simulink model "MyMotor_RTW"  (Simulink 10.1)
settings: Solver=ode1  StartTime=0.0  StopTime=inf  FixedStep=0.0002  RelTol=1e-3
PreLoadFcn:
  | vehicle = 'Car'; if ~length(which('cmcmd')), cmenv; end
  | MyMotor_RTW_bus
InitFcn:
  | vehicle = 'Car'; if ~length(which('cmcmd')), cmenv; end
  | MyMotor_RTW_bus
libraries: simulink x1, CarMaker4SL x1
Description:
  | CarMaker Plug-in Model Target
settings Model: Creator=ml  LastModifiedBy=ml
settings DataIOCC: LimitDataPoints=on  SignalLoggingSaveFormat=ModelDataLogs
settings OptimizationCC: ExpressionDepthLimit=2147483647
settings DebuggingCC: FcnCallInpInsideContextMsg=warning  StateNameClashWarn=warning  SFExecutionAtInitializationDiag=warning
settings HardwareCC: TargetHWDeviceType=32-bit Generic  ProdEqTarget=off
settings RTWCC: Description=CarMaker Plug-in Model Target  SystemTargetFile=CarMaker.tlc  TemplateMakefile=CarMaker_unix-win64.tmf
settings CodeAppCC: MaxIdLength=63
settings STFCustomTargetCC: ModelReferenceCompliant=off  MultiInstanceERTCode=on  CodeInterfacePackaging=Reusable function  CPPClassGenCompliant=on  GRTInterface=off  GenerateAllocFcn=on  SystemTargetFile=CarMaker.tlc
settings GRTTargetCC: ModelReferenceCompliant=off  ParMdlRefBuildCompliant=off  CompOptLevelCompliant=off  ConcurrentExecutionCompliant=off  MatFileLogging=off  MultiInstanceERTCode=on  CodeInterfacePackaging=Reusable function  GRTInterface=off  GenerateAllocFcn=on  UseToolchainInfoCompliant=off  ExtModeMexFile=noextcomm
settings CustomProperty: DataType=string
settings EnumStrPairs: String=Car

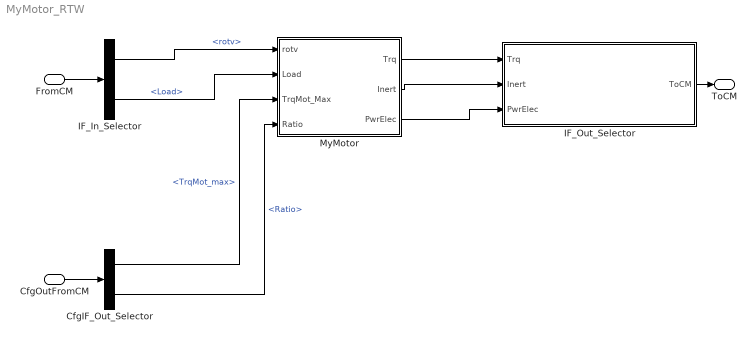
== system MyMotor_RTW ==
  FromCM : Inport  OutDataTypeStr=Bus: cmPTMotorIn
  CfgOutFromCM : Inport  Port=2  OutDataTypeStr=Bus: cmPTMotorCfgOut
  CfgIF_Out_Selector : BusSelector  OutputSignals=TrqMot_max,Ratio
  IF_In_Selector : BusSelector  OutputSignals=rotv,Load
  IF_Out_Selector : Subsystem  mask(Signal Selection){}
      mask help: Signal Selection Block
      settings: OpenFcn=cmSignalSelect('SignalSelection_CB',gcb)
  MyMotor : Subsystem
  ToCM : Outport  OutDataTypeStr=Bus: cmPTMotorOut  VectorParamsAs1DForOutWhenUnconnected=off
  wires:
  FromCM/1 -> IF_In_Selector/1
  IF_Out_Selector/1(ToCM) -> ToCM/1
  CfgOutFromCM/1 -> CfgIF_Out_Selector/1
  CfgIF_Out_Selector/1 -> MyMotor/3(TrqMot_Max)  "<TrqMot_max>"
  MyMotor/1(Trq) -> IF_Out_Selector/1(Trq)
  MyMotor/2(Inert) -> IF_Out_Selector/2(Inert)
  MyMotor/3(PwrElec) -> IF_Out_Selector/3(PwrElec)
  CfgIF_Out_Selector/2 -> MyMotor/4(Ratio)  "<Ratio>"
  IF_In_Selector/1 -> MyMotor/1(rotv)  "<rotv>"
  IF_In_Selector/2 -> MyMotor/2(Load)  "<Load>"

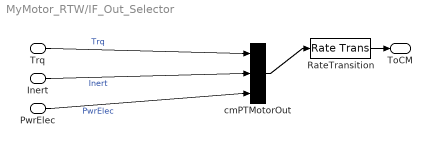
== system MyMotor_RTW/IF_Out_Selector ==
  Trq : Inport
  Inert : Inport  Port=2
  PwrElec : Inport  Port=3
  RateTransition : RateTransition  OutPortSampleTime=str2num(get_param(bdroot,'FixedStep'))
  cmPTMotorOut : BusCreator  Inputs=3
  ToCM : Outport  VectorParamsAs1DForOutWhenUnconnected=off
  wires:
  RateTransition/1 -> ToCM/1
  cmPTMotorOut/1 -> RateTransition/1
  Trq/1 -> cmPTMotorOut/1  "Trq"
  Inert/1 -> cmPTMotorOut/2  "Inert"
  PwrElec/1 -> cmPTMotorOut/3  "PwrElec"

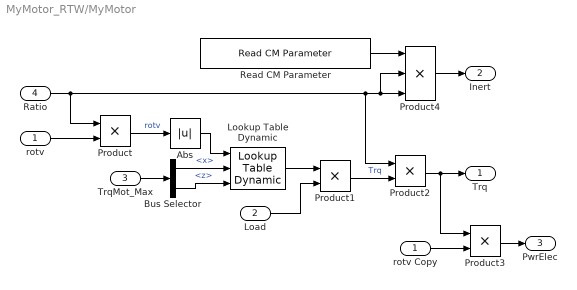
== system MyMotor_RTW/MyMotor ==
  rotv : Inport
  Load : Inport  Port=2
  TrqMot_Max : Inport  Port=3
  Ratio : Inport  Port=4
  Abs : Abs
  Bus Selector : BusSelector  OutputSignals=x,z
  Lookup Table Dynamic : simulink/Lookup Tables/Lookup Table Dynamic  LookUpMeth=Interpolation-Use End Values  OutDataTypeStr=float('double')  OutputDataTypeScalingMode=Specify via dialog  OutDataType=float('double')  OutScaling=2^-10  DoSatur=off
  Product{,1..3} (4 alike) : Product  RndMeth=Zero
  Product4 : Product  Inputs=3  RndMeth=Zero
  Read CM Parameter : CarMaker4SL/Read CM Parameter  xfile=Vehicle  xkey=PowerTrain.MotorISG.I  xnout=1  xdefaults=[]  xmuxed=on
      settings: SourceProductName=CarMaker4SL
  rotv Copy : InportShadow
  Trq : Outport  VectorParamsAs1DForOutWhenUnconnected=off
  Inert : Outport  Port=2  VectorParamsAs1DForOutWhenUnconnected=off
  PwrElec : Outport  Port=3  VectorParamsAs1DForOutWhenUnconnected=off
  wires:
  Ratio/1 -> Product2/1, Product4/3, Product4/2, Product/1
  Product/1 -> Abs/1  "rotv"
  TrqMot_Max/1 -> Bus Selector/1
  Bus Selector/1 -> Lookup Table Dynamic/2  "<x>"
  Bus Selector/2 -> Lookup Table Dynamic/3  "<z>"
  Abs/1 -> Lookup Table Dynamic/1
  Lookup Table Dynamic/1 -> Product1/1
  Load/1 -> Product1/2
  Product1/1 -> Product2/2  "Trq"
  Product2/1 -> Trq/1, Product3/1
  Product3/1 -> PwrElec/1
  Read CM Parameter/1 -> Product4/1
  Product4/1 -> Inert/1
  rotv Copy/1 -> Product3/2
  rotv/1 -> Product/2
